simulink model "lineal_integrator_lqr"  (R2024a)
settings: Solver=ode4  StartTime=0.0  StopTime=15  RelTol=1e-3
undefined symbols (not defined in the file or in its folder): DiscIntNeverNeededParam
libraries: simulink_extras x2
settings Model: Creator=Antón  LastModifiedBy=Antón
settings OptimizationCC: ZeroExternalMemoryAtStartup=off  ZeroInternalMemoryAtStartup=off
settings RTWCC: TargetLang=C++
settings GRTTargetCC: TargetLangStandard=C++11 (ISO)  CodeInterfacePackaging=C++ class

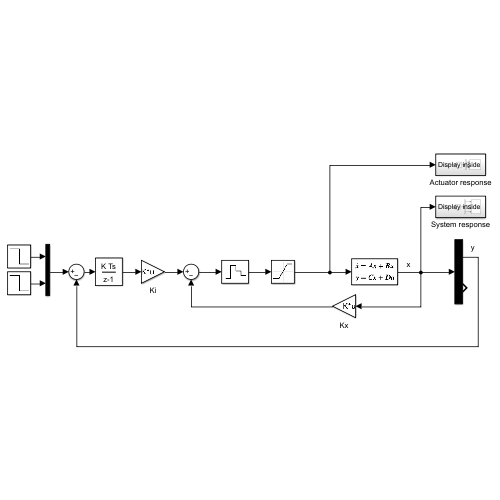
[thumbnail: Simulink's stored preview of the top-level diagram]
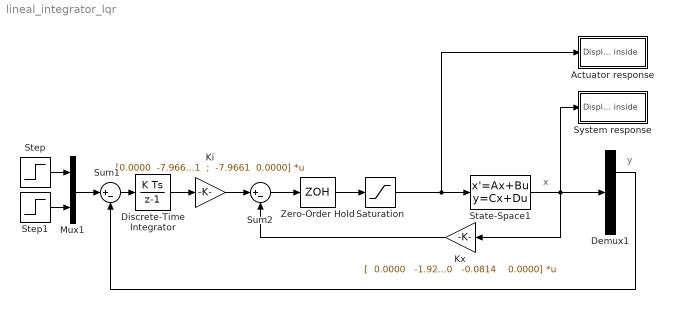
== system lineal_integrator_lqr ==
  note: x
  note: y
  Actuator response : Subsystem
  Demux1 : Demux  Outputs=2
  Discrete-Time Integrator : DiscreteIntegrator  SampleTime=-1  ICPrevOutput=DiscIntNeverNeededParam  ICPrevScaledInput=DiscIntNeverNeededParam
  Ki : Gain  Gain="[0.0000  -7.9661  ;  -7.9661  0.0000]"  Multiplication=Matrix(K*u)
  Kx : Gain  Gain="[  0.0000   -1.9285    0.0000   -0.0814 ;-1.9285   0.0000   -0.0814    0.0000]"  Multiplication=Matrix(K*u)
  Mux1 : Mux  Inputs=2
  Saturation : Saturate  UpperLimit=deg2rad(12)  LowerLimit=-deg2rad(12)
  State-Space1 : StateSpace  A=|  B=|  C=|  D=|  InitialCondition=0
      A=|
      | [0 0 1 0;
      |           0 0 0 1;
      |           0 0 0 0 ;
      |   0 0 0 0]
      B=|
      | [0  0;
      |           0 0 ;
      |           0 -535.9458;
      |   -535.9458  0]
      C=|
      | [1 0 0 0;
      |           0 1 0 0;
      |           0 0 1 0 ;
      |           0 0 0 1]
      D=|
      | [0  0;
      |           0 0;
      |           0 0 ;
      |           0 0]
  Step : Step  Time=7  Before=deg2rad(20)  After=0  SampleTime=0.02
  Step1 : Step  Time=10  Before=deg2rad(10)  After=0  SampleTime=0.02
  Sum1 : Sum  Inputs=|+-
  Sum2 : Sum  Inputs=|+-
  System response : Subsystem
  Zero-Order Hold : ZeroOrderHold  SampleTime=-1
  wires:
  Step1/1 -> Mux1/2
  Step/1 -> Mux1/1
  Kx/1 -> Sum2/2
  Sum1/1 -> Discrete-Time Integrator/1
  Discrete-Time Integrator/1 -> Ki/1
  Ki/1 -> Sum2/1
  Mux1/1 -> Sum1/1
  Sum2/1 -> Zero-Order Hold/1
  Saturation/1 -> Actuator response/1(Display inside), State-Space1/1
  Zero-Order Hold/1 -> Saturation/1
  State-Space1/1 -> Demux1/1, Kx/1, System response/1(Display inside)
  Demux1/1 -> Sum1/2

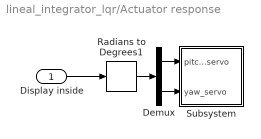
== system lineal_integrator_lqr/Actuator response ==
  Display inside : Inport
  Demux : Demux  Outputs=2
  Radians to Degrees1 : simulink_extras/Transformations/Radians to Degrees
  Subsystem : Subsystem
  wires:
  Radians to Degrees1/1 -> Demux/1
  Demux/1 -> Subsystem/1(pitch_servo)
  Demux/2 -> Subsystem/2(yaw_servo)
  Display inside/1 -> Radians to Degrees1/1

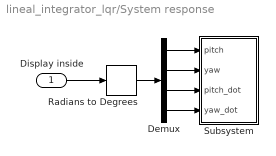
== system lineal_integrator_lqr/System response ==
  Display inside : Inport
  Demux : Demux
  Radians to Degrees : simulink_extras/Transformations/Radians to Degrees
  Subsystem : Subsystem
  wires:
  Radians to Degrees/1 -> Demux/1
  Display inside/1 -> Radians to Degrees/1
  Demux/3 -> Subsystem/3(pitch_dot)
  Demux/1 -> Subsystem/1(pitch)
  Demux/4 -> Subsystem/4(yaw_dot)
  Demux/2 -> Subsystem/2(yaw)

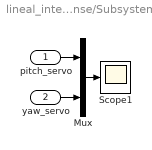
== system lineal_integrator_lqr/Actuator response/Subsystem ==
  pitch_servo : Inport
  yaw_servo : Inport  Port=2
  Mux : Mux  Inputs=2
  Scope1 : Scope
  wires:
  Mux/1 -> Scope1/1
  yaw_servo/1 -> Mux/2
  pitch_servo/1 -> Mux/1

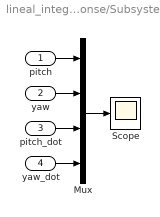
== system lineal_integrator_lqr/System response/Subsystem ==
  pitch : Inport
  yaw : Inport  Port=2
  pitch_dot : Inport  Port=3
  yaw_dot : Inport  Port=4
  Mux : Mux
  Scope : Scope
  wires:
  Mux/1 -> Scope/1
  pitch/1 -> Mux/1
  yaw/1 -> Mux/2
  pitch_dot/1 -> Mux/3
  yaw_dot/1 -> Mux/4
